simulink model "pid"  (R2025a)
settings: Solver=FixedStepAuto  StartTime=0.0  StopTime=10.0  FixedStep=1/50  RelTol=1e-3
settings Model: Creator=sucha  LastModifiedBy=sucha

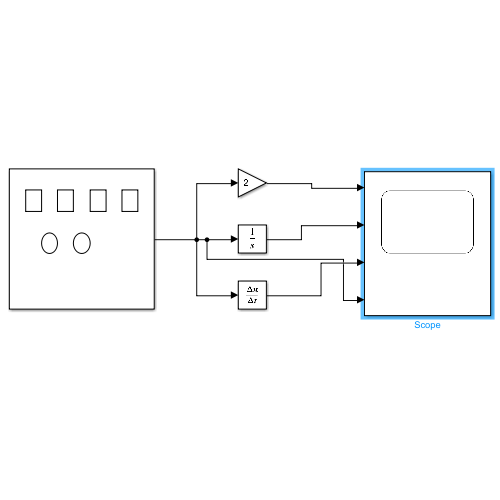
[thumbnail: Simulink's stored preview of the top-level diagram]
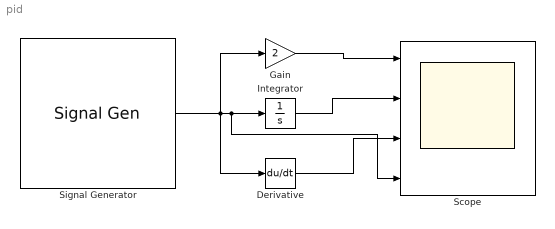
== system pid ==
  Derivative : Derivative
  Gain : Gain  Gain=2
  Integrator : Integrator
  Scope : Scope  NumInputPorts=4
      settings: ActiveDisplayYMinimum=-167.94360129729711  ActiveDisplayYMaximum=183.93542428383972
  Signal Generator : SignalGenerator  WaveForm=sawtooth  Amplitude=50  Frequency=.5
  wires:
  Signal Generator/1 -> Derivative/1, Scope/4, Integrator/1, Gain/1
  Gain/1 -> Scope/1
  Integrator/1 -> Scope/2
  Derivative/1 -> Scope/3
